simulink model "model3"  (R2024a)
settings: Solver=FixedStepAuto  StartTime=0.0  StopTime=36000  FixedStep=0.1  RelTol=1e-3
settings Model: Creator=rigel  LastModifiedBy=rigel

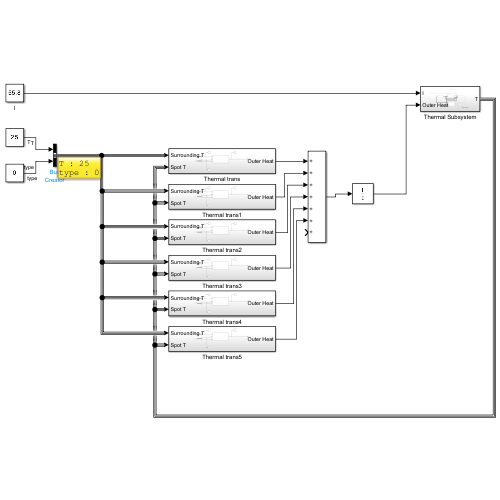
[thumbnail: Simulink's stored preview of the top-level diagram]
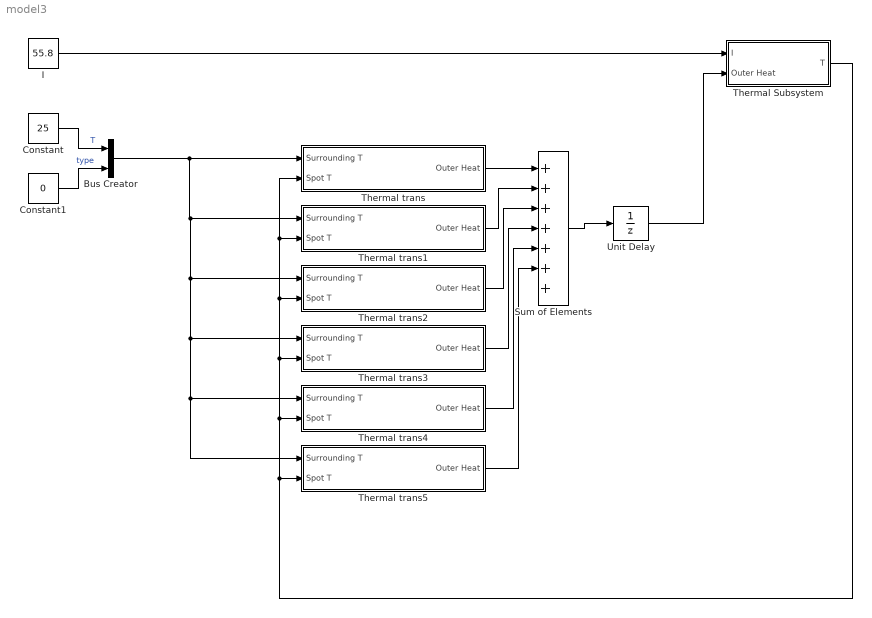
== system model3 ==
  Bus Creator : BusCreator  Inputs=2
  Constant : Constant  Value=25
  Constant1 : Constant  Value=0
  I : Constant  Value=55.8
  Sum of Elements : Sum  Inputs=+++++++
  Thermal Subsystem : Subsystem
  Thermal trans : Subsystem
  Thermal trans1 : Subsystem
  Thermal trans2 : Subsystem
  Thermal trans3 : Subsystem
  Thermal trans4 : Subsystem
  Thermal trans5 : Subsystem
  Unit Delay : UnitDelay  SampleTime=-1  HasFrameUpgradeWarning=on
  wires:
  Thermal Subsystem/1(T) -> Thermal trans/2(Spot T), Thermal trans1/2(Spot T), Thermal trans2/2(Spot T), Thermal trans3/2(Spot T), Thermal trans4/2(Spot T), Thermal trans5/2(Spot T)
  I/1 -> Thermal Subsystem/1(I)
  Unit Delay/1 -> Thermal Subsystem/2(Outer Heat)
  Constant/1 -> Bus Creator/1  "T"
  Constant1/1 -> Bus Creator/2  "type"
  Sum of Elements/1 -> Unit Delay/1
  Thermal trans/1(Outer Heat) -> Sum of Elements/1
  Thermal trans1/1(Outer Heat) -> Sum of Elements/2
  Thermal trans2/1(Outer Heat) -> Sum of Elements/3
  Thermal trans3/1(Outer Heat) -> Sum of Elements/4
  Thermal trans4/1(Outer Heat) -> Sum of Elements/5
  Thermal trans5/1(Outer Heat) -> Sum of Elements/6
  Bus Creator/1 -> Thermal trans5/1(Surrounding T), Thermal trans4/1(Surrounding T), Thermal trans3/1(Surrounding T), Thermal trans2/1(Surrounding T), Thermal trans1/1(Surrounding T), Thermal trans/1(Surrounding T)

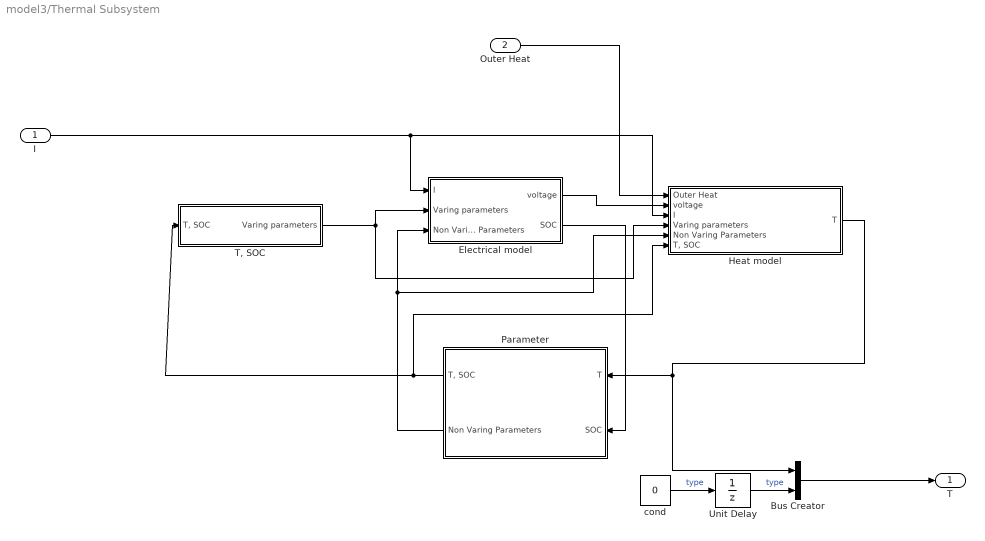
== system model3/Thermal Subsystem ==
  I : Inport
  Outer Heat : Inport  Port=2
  Bus Creator : BusCreator  Inputs=2
  Electrical model : Subsystem
  Heat model : Subsystem
  Parameter : Subsystem
  "T, SOC" : Subsystem
  Unit Delay : UnitDelay  SampleTime=-1  HasFrameUpgradeWarning=on
  cond : Constant  Value=0
  T : Outport
  wires:
  Parameter/2(Non Varing Parameters) -> Electrical model/3(Non Varing Parameters), Heat model/5(Non Varing Parameters)
  "T, SOC"/1(Varing parameters) -> Electrical model/2(Varing parameters), Heat model/4(Varing parameters)
  I/1 -> Heat model/3(I), Electrical model/1(I)
  Electrical model/2(SOC) -> Parameter/2(SOC)
  Electrical model/1(voltage) -> Heat model/2(voltage)
  Parameter/1("T, SOC") -> Heat model/6("T, SOC"), "T, SOC"/1("T, SOC")
  Outer Heat/1 -> Heat model/1(Outer Heat)
  Heat model/1(T) -> Bus Creator/1, Parameter/1(T)
  Bus Creator/1 -> T/1
  cond/1 -> Unit Delay/1  "type"
  Unit Delay/1 -> Bus Creator/2  "type"

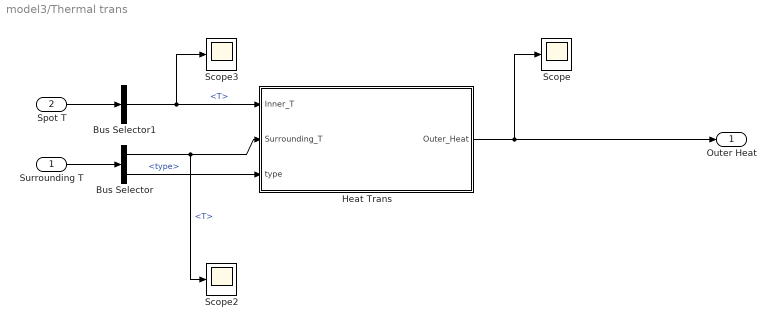
== system model3/Thermal trans ==
  Surrounding T : Inport
  Spot T : Inport  Port=2
  Bus Selector : BusSelector  OutputSignals=T,type
  Bus Selector1 : BusSelector  OutputSignals=T
  Heat Trans : MATLAB Function  TreatAsAtomicUnit=on
  Scope : Scope
  Scope2 : Scope
  Scope3 : Scope
  Outer Heat : Outport
  wires:
  Heat Trans/1(Outer_Heat) -> Scope/1, Outer Heat/1
  Bus Selector/1 -> Scope2/1, Heat Trans/2(Surrounding_T)  "<T>"
  Bus Selector/2 -> Heat Trans/3(type)  "<type>"
  Bus Selector1/1 -> Scope3/1, Heat Trans/1(Inner_T)  "<T>"
  Spot T/1 -> Bus Selector1/1
  Surrounding T/1 -> Bus Selector/1

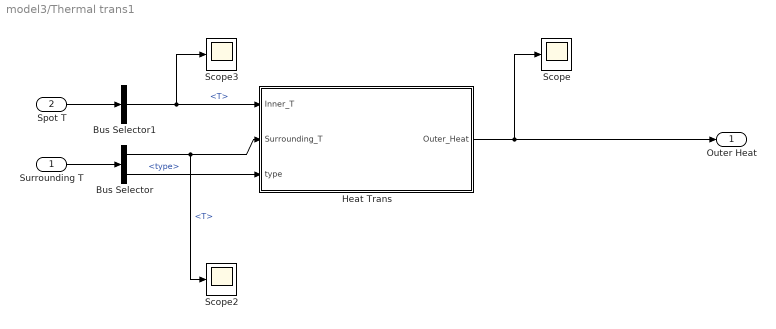
== system model3/Thermal trans1 ==
  Surrounding T : Inport
  Spot T : Inport  Port=2
  Bus Selector : BusSelector  OutputSignals=T,type
  Bus Selector1 : BusSelector  OutputSignals=T
  Heat Trans : MATLAB Function  TreatAsAtomicUnit=on
  Scope : Scope
  Scope2 : Scope
  Scope3 : Scope
  Outer Heat : Outport
  wires:
  Heat Trans/1(Outer_Heat) -> Scope/1, Outer Heat/1
  Bus Selector/1 -> Scope2/1, Heat Trans/2(Surrounding_T)  "<T>"
  Bus Selector/2 -> Heat Trans/3(type)  "<type>"
  Bus Selector1/1 -> Scope3/1, Heat Trans/1(Inner_T)  "<T>"
  Spot T/1 -> Bus Selector1/1
  Surrounding T/1 -> Bus Selector/1

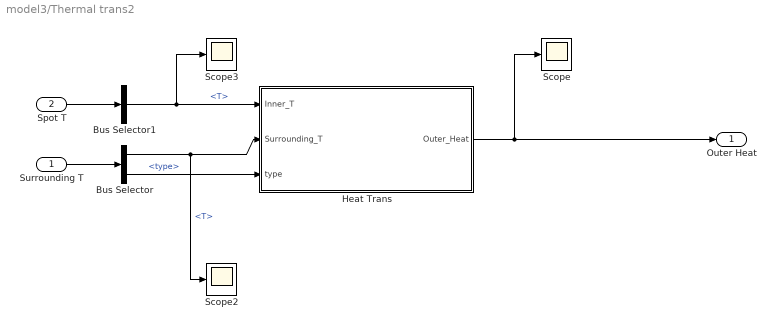
== system model3/Thermal trans2 ==
  Surrounding T : Inport
  Spot T : Inport  Port=2
  Bus Selector : BusSelector  OutputSignals=T,type
  Bus Selector1 : BusSelector  OutputSignals=T
  Heat Trans : MATLAB Function  TreatAsAtomicUnit=on
  Scope : Scope
  Scope2 : Scope
  Scope3 : Scope
  Outer Heat : Outport
  wires:
  Heat Trans/1(Outer_Heat) -> Scope/1, Outer Heat/1
  Bus Selector/1 -> Scope2/1, Heat Trans/2(Surrounding_T)  "<T>"
  Bus Selector/2 -> Heat Trans/3(type)  "<type>"
  Bus Selector1/1 -> Scope3/1, Heat Trans/1(Inner_T)  "<T>"
  Spot T/1 -> Bus Selector1/1
  Surrounding T/1 -> Bus Selector/1

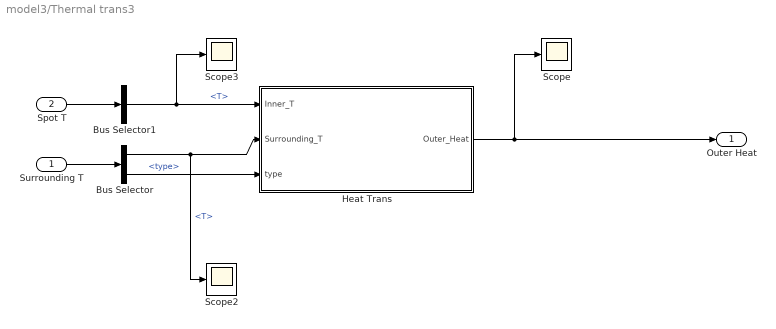
== system model3/Thermal trans3 ==
  Surrounding T : Inport
  Spot T : Inport  Port=2
  Bus Selector : BusSelector  OutputSignals=T,type
  Bus Selector1 : BusSelector  OutputSignals=T
  Heat Trans : MATLAB Function  TreatAsAtomicUnit=on
  Scope : Scope
  Scope2 : Scope
  Scope3 : Scope
  Outer Heat : Outport
  wires:
  Heat Trans/1(Outer_Heat) -> Scope/1, Outer Heat/1
  Bus Selector/1 -> Scope2/1, Heat Trans/2(Surrounding_T)  "<T>"
  Bus Selector/2 -> Heat Trans/3(type)  "<type>"
  Bus Selector1/1 -> Scope3/1, Heat Trans/1(Inner_T)  "<T>"
  Spot T/1 -> Bus Selector1/1
  Surrounding T/1 -> Bus Selector/1

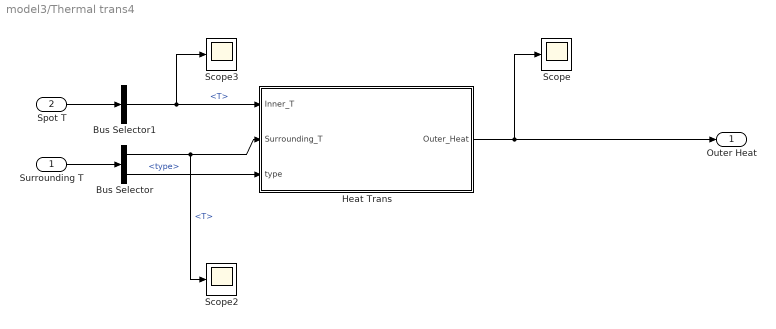
== system model3/Thermal trans4 ==
  Surrounding T : Inport
  Spot T : Inport  Port=2
  Bus Selector : BusSelector  OutputSignals=T,type
  Bus Selector1 : BusSelector  OutputSignals=T
  Heat Trans : MATLAB Function  TreatAsAtomicUnit=on
  Scope : Scope
  Scope2 : Scope
  Scope3 : Scope
  Outer Heat : Outport
  wires:
  Heat Trans/1(Outer_Heat) -> Scope/1, Outer Heat/1
  Bus Selector/1 -> Scope2/1, Heat Trans/2(Surrounding_T)  "<T>"
  Bus Selector/2 -> Heat Trans/3(type)  "<type>"
  Bus Selector1/1 -> Scope3/1, Heat Trans/1(Inner_T)  "<T>"
  Spot T/1 -> Bus Selector1/1
  Surrounding T/1 -> Bus Selector/1

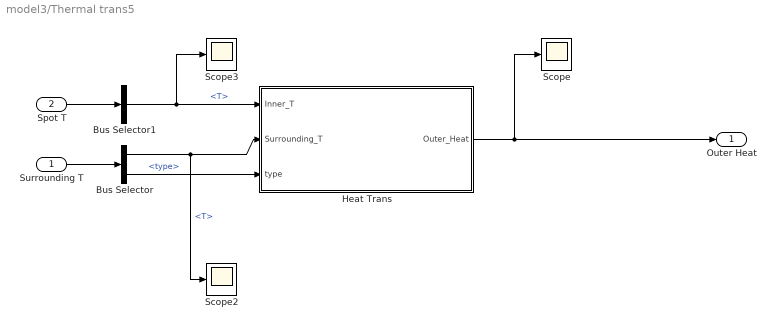
== system model3/Thermal trans5 ==
  Surrounding T : Inport
  Spot T : Inport  Port=2
  Bus Selector : BusSelector  OutputSignals=T,type
  Bus Selector1 : BusSelector  OutputSignals=T
  Heat Trans : MATLAB Function  TreatAsAtomicUnit=on
  Scope : Scope
  Scope2 : Scope
  Scope3 : Scope
  Outer Heat : Outport
  wires:
  Heat Trans/1(Outer_Heat) -> Scope/1, Outer Heat/1
  Bus Selector/1 -> Scope2/1, Heat Trans/2(Surrounding_T)  "<T>"
  Bus Selector/2 -> Heat Trans/3(type)  "<type>"
  Bus Selector1/1 -> Scope3/1, Heat Trans/1(Inner_T)  "<T>"
  Spot T/1 -> Bus Selector1/1
  Surrounding T/1 -> Bus Selector/1

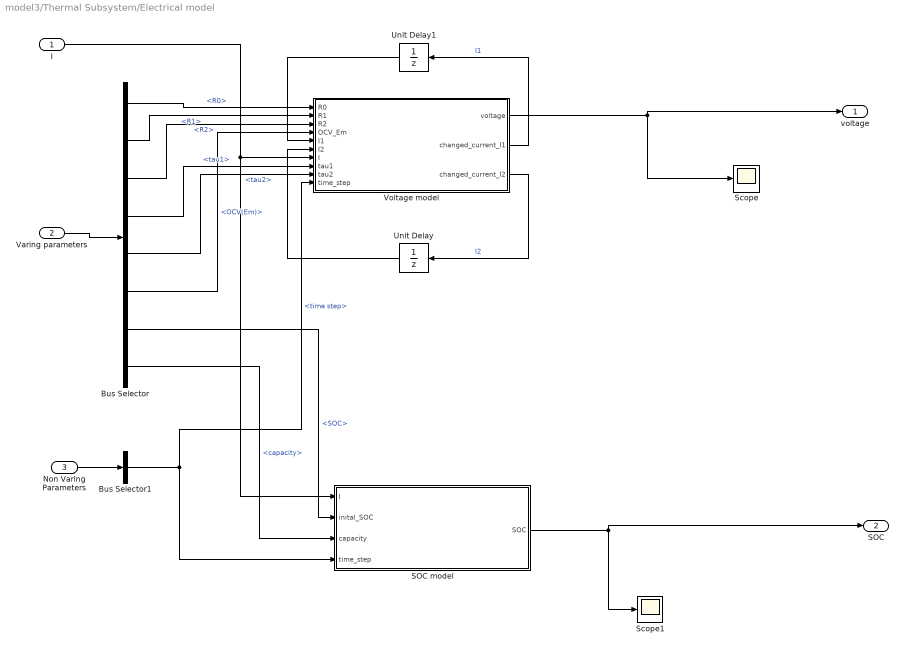
== system model3/Thermal Subsystem/Electrical model ==
  I : Inport
  Varing parameters : Inport  Port=2
  Non Varing Parameters : Inport  Port=3
  Bus Selector : BusSelector  OutputSignals=R0,R1,R2,tau1,tau2,OCV(Em),SOC,capacity
  Bus Selector1 : BusSelector  OutputSignals=time step
  SOC model : MATLAB Function  TreatAsAtomicUnit=on
  Scope : Scope
  Scope1 : Scope
  Unit Delay : UnitDelay  SampleTime=-1  HasFrameUpgradeWarning=on
  Unit Delay1 : UnitDelay  SampleTime=-1  HasFrameUpgradeWarning=on
  Voltage model : MATLAB Function  TreatAsAtomicUnit=on
  voltage : Outport
  SOC : Outport  Port=2
  wires:
  Varing parameters/1 -> Bus Selector/1
  Bus Selector/1 -> Voltage model/1(R0)  "<R0>"
  Bus Selector/2 -> Voltage model/2(R1)  "<R1>"
  Bus Selector/3 -> Voltage model/3(R2)  "<R2>"
  Bus Selector/4 -> Voltage model/8(tau1)  "<tau1>"
  Bus Selector/5 -> Voltage model/9(tau2)  "<tau2>"
  Bus Selector/6 -> Voltage model/4(OCV_Em)  "<OCV(Em)>"
  SOC model/1(SOC) -> SOC/1, Scope1/1
  Voltage model/1(voltage) -> voltage/1, Scope/1
  I/1 -> SOC model/1(I), Voltage model/7(I)
  Voltage model/2(changed_current_I1) -> Unit Delay1/1  "I1"
  Unit Delay1/1 -> Voltage model/5(I1)
  Voltage model/3(changed_current_I2) -> Unit Delay/1  "I2"
  Unit Delay/1 -> Voltage model/6(I2)
  Bus Selector/7 -> SOC model/2(inital_SOC)  "<SOC>"
  Non Varing Parameters/1 -> Bus Selector1/1
  Bus Selector1/1 -> Voltage model/10(time_step), SOC model/4(time_step)  "<time step>"
  Bus Selector/8 -> SOC model/3(capacity)  "<capacity>"

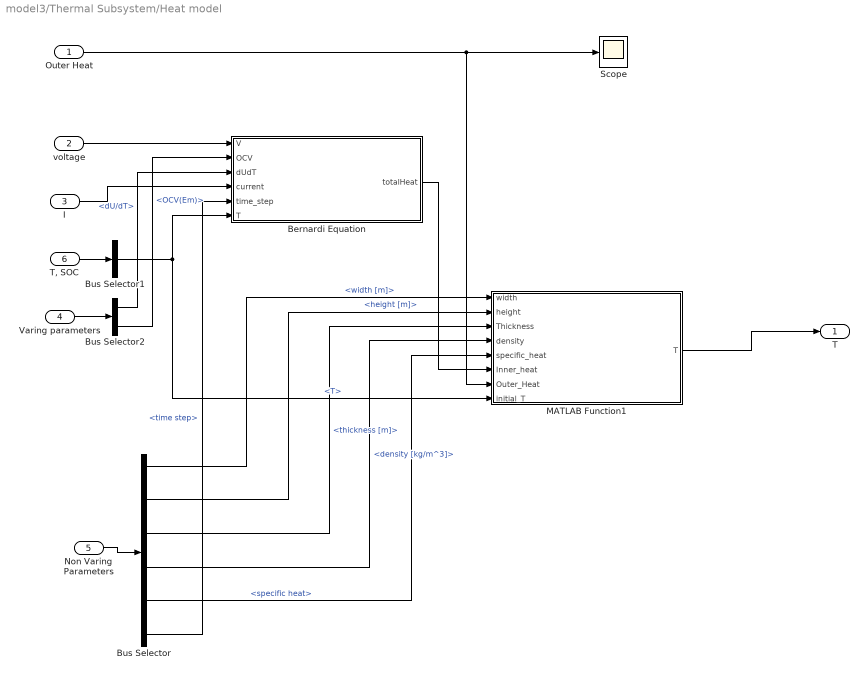
== system model3/Thermal Subsystem/Heat model ==
  Outer Heat : Inport
  voltage : Inport  Port=2
  I : Inport  Port=3
  Varing parameters : Inport  Port=4
  Non Varing Parameters : Inport  Port=5
  "T, SOC" : Inport  Port=6
  Bernardi Equation : MATLAB Function  TreatAsAtomicUnit=on
  Bus Selector : BusSelector  OutputSignals=width [m],height [m],thickness [m],density [kg/m^3],specific heat,time step
  Bus Selector1 : BusSelector  OutputSignals=T
  Bus Selector2 : BusSelector  OutputSignals=dU/dT,OCV(Em)
  MATLAB Function1 : MATLAB Function  TreatAsAtomicUnit=on
  Scope : Scope
  T : Outport
  wires:
  voltage/1 -> Bernardi Equation/1(V)
  MATLAB Function1/1(T) -> T/1
  Bernardi Equation/1(totalHeat) -> MATLAB Function1/6(Inner_heat)
  Non Varing Parameters/1 -> Bus Selector/1
  Bus Selector/1 -> MATLAB Function1/1(width)  "<width [m]>"
  Bus Selector/2 -> MATLAB Function1/2(height)  "<height [m]>"
  Bus Selector/3 -> MATLAB Function1/3(Thickness)  "<thickness [m]>"
  Bus Selector/4 -> MATLAB Function1/4(density)  "<density [kg/m^3]>"
  Bus Selector/5 -> MATLAB Function1/5(specific_heat)  "<specific heat>"
  "T, SOC"/1 -> Bus Selector1/1
  Bus Selector1/1 -> MATLAB Function1/8(initial_T), Bernardi Equation/6(T)  "<T>"
  I/1 -> Bernardi Equation/4(current)
  Varing parameters/1 -> Bus Selector2/1
  Bus Selector2/1 -> Bernardi Equation/3(dUdT)  "<dU/dT>"
  Bus Selector2/2 -> Bernardi Equation/2(OCV)  "<OCV(Em)>"
  Bus Selector/6 -> Bernardi Equation/5(time_step)  "<time step>"
  Outer Heat/1 -> MATLAB Function1/7(Outer_Heat), Scope/1

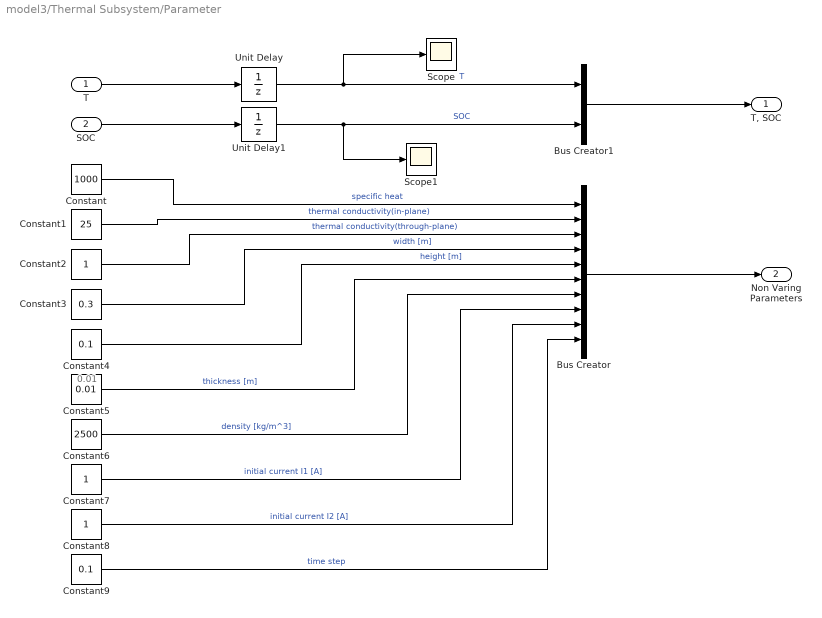
== system model3/Thermal Subsystem/Parameter ==
  note: 0.01
  T : Inport
  SOC : Inport  Port=2
  Bus Creator : BusCreator  Inputs=10
  Bus Creator1 : BusCreator  Inputs=2
  Constant : Constant  Value=1000
  Constant1 : Constant  Value=25
  Constant2 : Constant
  Constant3 : Constant  Value=0.3
  Constant4 : Constant  Value=0.1
  Constant5 : Constant  Value=0.01
  Constant6 : Constant  Value=2500
  Constant7 : Constant
  Constant8 : Constant
  Constant9 : Constant  Value=0.1
  Scope : Scope
  Scope1 : Scope
  Unit Delay : UnitDelay  InitialCondition=25  HasFrameUpgradeWarning=on
  Unit Delay1 : UnitDelay  InitialCondition=1  HasFrameUpgradeWarning=on
  "T, SOC" : Outport
  Non Varing Parameters : Outport  Port=2
  wires:
  Constant2/1 -> Bus Creator/3  "thermal conductivity(through-plane)"
  Constant/1 -> Bus Creator/1  "specific heat"
  Constant8/1 -> Bus Creator/9  "initial current I2 [A]"
  Constant6/1 -> Bus Creator/7  "density [kg/m^3]"
  Constant5/1 -> Bus Creator/6  "thickness [m]"
  Constant1/1 -> Bus Creator/2  "thermal conductivity(in-plane)"
  Constant4/1 -> Bus Creator/5  "height [m]"
  Constant7/1 -> Bus Creator/8  "initial current I1 [A]"
  Constant3/1 -> Bus Creator/4  "width [m]"
  Unit Delay/1 -> Scope/1, Bus Creator1/1  "T"
  Unit Delay1/1 -> Scope1/1, Bus Creator1/2  "SOC"
  T/1 -> Unit Delay/1
  SOC/1 -> Unit Delay1/1
  Bus Creator1/1 -> "T, SOC"/1
  Bus Creator/1 -> Non Varing Parameters/1
  Constant9/1 -> Bus Creator/10  "time step"

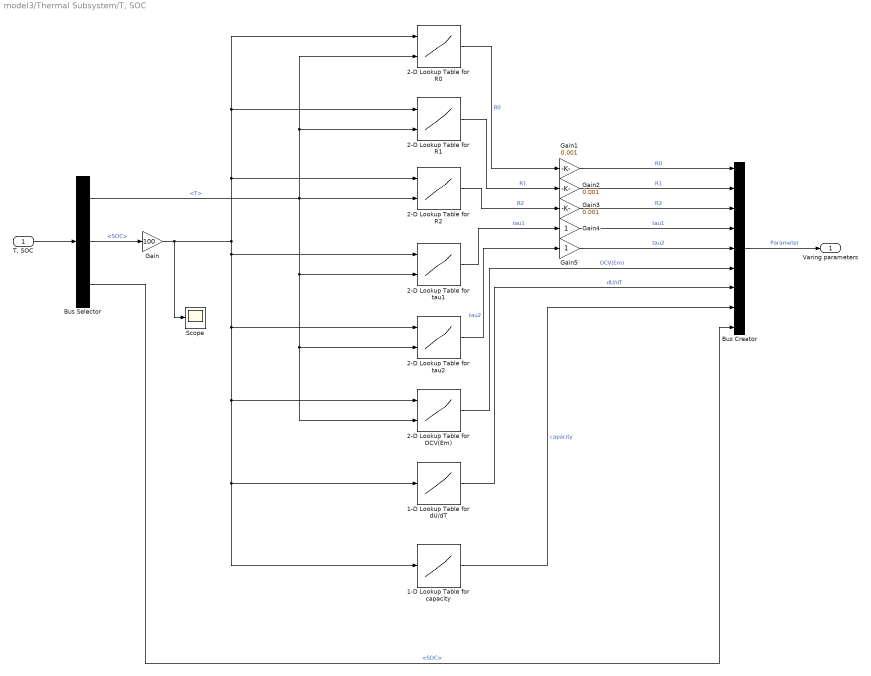
== system model3/Thermal Subsystem/T, SOC ==
  "T, SOC" : Inport
  1-D Lookup Table for capacity : Lookup_n-D  NumberOfTableDimensions=1  BreakpointsForDimension1=[5;15;25;35;45]  Table=[51.8;54.3;55.8;57.2;57.3]  InternalRulePriority=Speed  RndMeth=Simplest
  1-D Lookup Table for dU/dT : Lookup_n-D  NumberOfTableDimensions=1  BreakpointsForDimension1=[0 10 20 30 40 50 60 70 80 90 100]  Table=[-0.0004 -9e-05 -3e-05 9e-05 0.00016 9e-05 5e-05 5e-05 6e-05 9e-05 8e-05]  InternalRulePriority=Speed  RndMeth=Simplest
  2-D Lookup Table for OCV(Em) : Lookup_n-D  BreakpointsForDimension1=[0;2.5;4.987882;7.488427;9.988971;14.98952;19.99007;24.99062;29.99118;34.99173;39.99229;44.99284;49.9934;54.99394;59.99449;64.99504;69.99559;74.99614;79.99669;84.99724;89.99779;92.49834;94.9989;97.49945;100]  BreakpointsForDimension2=[5 15 25 35 45]  Table=[3.41 3.37 3.23 3.23 3.23;3.43 3.4 3.36 3.36 3.36;3.45 3.42 3.4 3.41 3.41;3.48 3.44 3.42 3.43 3.43;3.51 3.47 3.44 3.45 3.45;3.55 3.52 3.5 3.5 3.5;3.58 3.56 3.54 3.55 3.55;3.6 3.59 3.58 3.58 3.58;3.61 3.61 3.6 3.61 3.61;3.63 3.63 3.62 3.62 3.62;3.65 3.65 3.64 3.64 3.64;3.68 3.67 3.66 3.67 3.67;3.72 3.71 3.7 3.7 3.7;3.78 3.77 3.75 3.76 3.76;3.83 3.82 3.81 3.81 3.81;3.87 3.86 3.85 3.86 3.86;3.91 3.9 3.89 3.9 3.9;3.94 3.94 3.93 3.94 3.94;4 3.99 3.98 3.99 3.99;4.04 4.04 4.03 4.04 4.04;4.07 4.08 4.07 4.08 4.08;4.08 4.09 4.09 4.09 4.09;4.1 4.1 4.1 4.11 4.11;4.12 4.13 4.13 4.14 4.14;4.17 4.18 4.18 4.19 4.19]  InternalRulePriority=Speed  RndMeth=Simplest
      settings: InputPortMap=u0,u1
  2-D Lookup Table for R0 : Lookup_n-D  BreakpointsForDimension1=[4.987882;7.488427;9.988971;14.98952;19.99007;24.99062;29.99118;34.99173;39.99229;44.99284;49.9934;54.99394;59.99449;64.99504;69.99559;74.99614;79.99669;84.99724;89.99779;92.49834;94.9989;97.49945;100]  BreakpointsForDimension2=[5 15 25 35 45]  Table=[2.5 1.660027 1.399329 1 0.85;2.5 1.567803 1.309628 0.95 0.8;2 1.512469 1.237868 0.9 0.75;2 1.383279 1.130227 0.8 0.7;2 1.291108 1.058467 0.75 0.7;1.75 1.235729 1 0.75 0.65;1.75 1.217285 0.95 0.75 0.65;1.75 1.198842 0.95 0.75 0.65;1.75 1.180398 0.95 0.75 0.65;1.75 1.161954 0.95 0.75 0.65;1.75 1.161954 0.95 0.75 0.65;1.5 1.2 0.95 0.7 0.65;1.5 1.2 0.95 0.7 0.65;1.5 1.2 0.95 0.7 0.65;1.5 1.2 0.95 0.7 0.65;1.5 1.2 0.95 0.7 0.65;1.5 1.2 0.95 0.7 0.65;1.75 1.2 0.95 0.75 0.65;1.75 1.180398 0.95 0.75 0.65;1.75 1.198842 0.95 0.75 0.65;2 1.217353 1 0.75 0.65;2 1.235798 1 0.75 0.65;2 1.235798 1 0.75 0.65]  InternalRulePriority=Speed  RndMeth=Simplest
      settings: InputPortMap=u0,u1
  2-D Lookup Table for R1 : Lookup_n-D  BreakpointsForDimension1=[4.987882;7.488427;9.988971;14.98952;19.99007;24.99062;29.99118;34.99173;39.99229;44.99284;49.9934;54.99394;59.99449;64.99504;69.99559;74.99614;79.99669;84.99724;89.99779;92.49834;94.9989;97.49945;100]  BreakpointsForDimension2=[5 15 25 35 45]  Table=[1.343459 1 0.95 0.55 0.4;0.95 0.65 0.65 0.55 0.4;0.7 0.5 0.5 0.45 0.4;0.45 0.4 0.4 0.35 0.35;0.45 0.4 0.4 0.3 0.3;0.4 0.35 0.4 0.3 0.3;0.4 0.4 0.4 0.3 0.3;0.4 0.3 0.4 0.3 0.3;0.35 0.3 0.4 0.3 0.3;0.35 0.3 0.4 0.3 0.3;0.45 0.35 0.4 0.3 0.3;0.5 0.45 0.45 0.35 0.3;0.55 0.5 0.45 0.35 0.3;0.45 0.4 0.4 0.35 0.35;0.45 0.4 0.4 0.35 0.35;0.45 0.4 0.4 0.35 0.3;0.5 0.4 0.4 0.35 0.3;0.45 0.4 0.35 0.25 0.25;0.4 0.35 0.35 0.25 0.25;0.4 0.35 0.35 0.3 0.25;0.45 0.4 0.3 0.25 0.25;0.45 0.45 0.35 0.35 0.25;0.5 0.45 0.4 0.35 0.3]  InternalRulePriority=Speed  RndMeth=Simplest
      settings: InputPortMap=u0,u1
  2-D Lookup Table for R2 : Lookup_n-D  BreakpointsForDimension1=[4.987882;7.488427;9.988971;14.98952;19.99007;24.99062;29.99118;34.99173;39.99229;44.99284;49.9934;54.99394;59.99449;64.99504;69.99559;74.99614;79.99669;84.99724;89.99779;92.49834;94.9989;97.49945;100]  BreakpointsForDimension2=[5 15 25 35 45]  Table=[11.25 10 8 6.3 5.062057;4 3.773492 4.3 2.7 1.418744;3 1.926279 2.088626 1.5 1;2.75 1.741972 1.371574 0.8 0.65;2.5 1.58323 1.235492 0.8 0.65;2 1.585742 1.227908 0.8 0.65;1.75 1.41798 1.3 0.9 0.65;1.75 1.19079 1.090479 0.9 0.65;1.5 1 0.9 0.7 0.7;1.5 0.9 0.9 0.7 0.6;1.5 0.9 0.9 0.7 0.6;1.5 0.9 0.9 0.7 0.6;1.5 1 1 0.8 0.65;1.504995 1.233499 1.1 0.9 0.75;1.47432 1.196612 1 0.8 0.7;1.5 1.138683 0.95 0.75 0.65;1.25 1 0.9 0.7 0.55;1.25 1 0.85 0.6 0.45;1.25 0.9 0.7 0.55 0.4;1 0.8 0.75 0.5 0.4;0.9 0.7 0.6 0.4 0.3;0.9 0.6 0.55 0.4 0.3;1 0.7 0.6 0.4 0.35]  InternalRulePriority=Speed  RndMeth=Simplest
      settings: InputPortMap=u0,u1
  2-D Lookup Table for tau1 : Lookup_n-D  BreakpointsForDimension1=[4.987882;7.488427;9.988971;14.98952;19.99007;24.99062;29.99118;34.99173;39.99229;44.99284;49.9934;54.99394;59.99449;64.99504;69.99559;74.99614;79.99669;84.99724;89.99779;92.49834;94.9989;97.49945;100]  BreakpointsForDimension2=[5 15 25 35 45]  Table=[1.15 1.5 1.96 3.39 3.09;1.25 1.9 2.8 5.27 3.89;1.6 2.3 3.03 5.23 4.07;2.15 3.6 3.65 4.14 4.77;3.35 5.4 5.35 4.55 4.53;3.85 4.1 4.83 3.83 3.53;4.35 6.4 4.6 5.36 3.61;5.15 4.1 4.45 3.75 3.21;4.3 4 5.49 4.61 3.54;3.65 4.3 3.94 3.53 3.71;4.4 4.1 5.2 3.76 2.99;4.55 5.1 5.38 3.7 3.53;4.7 5.8 4.82 4.14 3.43;3.8 4.3 3.59 3.48 4.16;3.7 4.5 4.02 4.38 4.31;3.95 4.4 4.67 4.46 4.07;4.9 4.7 4.09 3.92 3.73;4.5 4.4 4.26 3.1 2.93;3.5 4.4 4.47 3.66 3.47;3.8 3.6 4.29 3.85 2.77;3.5 4.6 3.44 2.98 2.89;3.45 4.8 3.92 4.27 3.32;3.4 4.2 4.42 4.16 3.92]  InternalRulePriority=Speed  RndMeth=Simplest
      settings: InputPortMap=u0,u1
  2-D Lookup Table for tau2 : Lookup_n-D  BreakpointsForDimension1=[4.987882;7.488427;9.988971;14.98952;19.99007;24.99062;29.99118;34.99173;39.99229;44.99284;49.9934;54.99394;59.99449;64.99504;69.99559;74.99614;79.99669;84.99724;89.99779;92.49834;94.9989;97.49945;100]  BreakpointsForDimension2=[5 15 25 35 45]  Table=[185 300 300 93.67 300;75.3 91.2 148.77 105.74 77.83;67.8 53.3 66.88 56.32 53.02;85.4 70.7 59.61 43.37 45.34;86.5 85.4 71.75 54.67 41.7;78.9 75.8 71.19 50.7 40.55;71.8 87.8 71.96 73.22 46.89;66.1 60.7 63.92 57.62 54.37;52.2 52.1 64.06 53.52 48.88;44.6 47.1 47.41 40.53 42.49;41.1 37.4 46.1 35.98 35.33;36.8 31.7 31.79 22.48 20.07;46.1 45.9 37.76 36.57 27;47.9 46.8 41.38 39.18 38.88;49.4 49.4 46.03 44.18 41.55;49.3 48.9 49.79 43.32 38.38;52.3 46.5 43.5 38.44 34.2;53.4 49.7 46.26 35.85 31.25;52.6 54.4 51.32 46.11 41.98;49.6 44.3 54.68 46.3 43.67;36.3 40.6 33.94 25.83 34.83;31.6 33.5 27.37 26.04 19.14;30.3 31.5 29.11 25.72 22.48]  InternalRulePriority=Speed  RndMeth=Simplest
      settings: InputPortMap=u0,u1
  Bus Creator : BusCreator  Inputs=9
  Bus Selector : BusSelector  OutputSignals=T,SOC,SOC
  Gain : Gain  Gain=100
  Gain1 : Gain  Gain=0.001
  Gain2 : Gain  Gain=0.001
  Gain3 : Gain  Gain=0.001
  Gain4 : Gain
  Gain5 : Gain
  Scope : Scope
  Varing parameters : Outport
  wires:
  2-D Lookup Table for OCV(Em)/1 -> Bus Creator/6  "OCV(Em)"
  2-D Lookup Table for tau2/1 -> Gain5/1  "tau2"
  2-D Lookup Table for R2/1 -> Gain3/1  "R2"
  2-D Lookup Table for tau1/1 -> Gain4/1  "tau1"
  2-D Lookup Table for R0/1 -> Gain1/1  "R0"
  2-D Lookup Table for R1/1 -> Gain2/1  "R1"
  Bus Creator/1 -> Varing parameters/1  "Parameter"
  1-D Lookup Table for dU/dT/1 -> Bus Creator/7  "dU/dT"
  "T, SOC"/1 -> Bus Selector/1
  Bus Selector/1 -> 2-D Lookup Table for OCV(Em)/2, 2-D Lookup Table for tau2/2, 2-D Lookup Table for tau1/2, 2-D Lookup Table for R2/2, 2-D Lookup Table for R1/2, 2-D Lookup Table for R0/2  "<T>"
  Bus Selector/3 -> Bus Creator/9  "<SOC>"
  Bus Selector/2 -> Gain/1  "<SOC>"
  Gain/1 -> 2-D Lookup Table for R1/1, 2-D Lookup Table for R0/1, 2-D Lookup Table for R2/1, 2-D Lookup Table for tau2/1, 2-D Lookup Table for OCV(Em)/1, 1-D Lookup Table for dU/dT/1, 1-D Lookup Table for capacity/1, 2-D Lookup Table for tau1/1, Scope/1
  1-D Lookup Table for capacity/1 -> Bus Creator/8  "capacity"
  Gain1/1 -> Bus Creator/1  "R0"
  Gain2/1 -> Bus Creator/2  "R1"
  Gain3/1 -> Bus Creator/3  "R2"
  Gain4/1 -> Bus Creator/4  "tau1"
  Gain5/1 -> Bus Creator/5  "tau2"

== matlab function model3/Thermal trans4/Heat Trans ==
  data: Inner_T input; Outer_Heat output; Surrounding_T input; type input
function Outer_Heat = fcn(Inner_T, Surrounding_T, type)
%#codegen
% Inputs
%   Inner_T        : 내부 온도 (scalar)
%   Surrounding    : struct with fields
%       .T         : 주변 온도
%       .mode      : 0 = conduction, 1 = convection

k = 1;    % 열전도도 (W/(m·K))
A = 0.01;    % 면적 (m^2)
L = 0.1;    % 길이 (m)
h = 1;    % 대류 열전달계수 (W/(m^2·K))

G_cond = k * A / L;      % 전도 전도도 (W/K)
G_conv = h * A;          % 대류 전도도   (W/K)

if type == 0
    % 전도
    % q = G_cond * (ΔT)
    Outer_Heat = - G_cond * (Inner_T - Surrounding_T);
elseif type == 1
    % 대류
    % q = G_conv * (ΔT)
    Outer_Heat = - G_conv * (Inner_T - Surrounding_T);
else
    % 정의되지 않은 모드일 때
    Outer_Heat = 0;
end

== matlab function model3/Thermal trans5/Heat Trans ==
  data: Inner_T input; Outer_Heat output; Surrounding_T input; type input
function Outer_Heat = fcn(Inner_T, Surrounding_T, type)
%#codegen
% Inputs
%   Inner_T        : 내부 온도 (scalar)
%   Surrounding    : struct with fields
%       .T         : 주변 온도
%       .mode      : 0 = conduction, 1 = convection

k = 1;    % 열전도도 (W/(m·K))
A = 0.01;    % 면적 (m^2)
L = 0.1;    % 길이 (m)
h = 1;    % 대류 열전달계수 (W/(m^2·K))

G_cond = k * A / L;      % 전도 전도도 (W/K)
G_conv = h * A;          % 대류 전도도   (W/K)

if type == 0
    % 전도
    % q = G_cond * (ΔT)
    Outer_Heat = - G_cond * (Inner_T - Surrounding_T);
elseif type == 1
    % 대류
    % q = G_conv * (ΔT)
    Outer_Heat = - G_conv * (Inner_T - Surrounding_T);
else
    % 정의되지 않은 모드일 때
    Outer_Heat = 0;
end

== matlab function model3/Thermal trans/Heat Trans ==
  data: Inner_T input; Outer_Heat output; Surrounding_T input; type input
function Outer_Heat = fcn(Inner_T, Surrounding_T, type)
%#codegen
% Inputs
%   Inner_T        : 내부 온도 (scalar)
%   Surrounding    : struct with fields
%       .T         : 주변 온도
%       .mode      : 0 = conduction, 1 = convection

k = 1;    % 열전도도 (W/(m·K))
A = 0.01;    % 면적 (m^2)
L = 0.1;    % 길이 (m)
h = 1;    % 대류 열전달계수 (W/(m^2·K))

G_cond = k * A / L;      % 전도 전도도 (W/K)
G_conv = h * A;          % 대류 전도도   (W/K)

if type == 0
    % 전도
    % q = G_cond * (ΔT)
    Outer_Heat = - G_cond * (Inner_T - Surrounding_T);
elseif type == 1
    % 대류
    % q = G_conv * (ΔT)
    Outer_Heat = - G_conv * (Inner_T - Surrounding_T);
else
    % 정의되지 않은 모드일 때
    Outer_Heat = 0;
end

== matlab function model3/Thermal Subsystem/Electrical model/SOC model ==
  data: SOC output; I input; inital_SOC input; capacity input; time_step input
function SOC = fcn(I, inital_SOC, capacity, time_step)
    % Cn = 55.8 * 3600;
    SOC = inital_SOC - (I * time_step / (capacity * 3600));
end

== matlab function model3/Thermal Subsystem/Electrical model/Voltage model ==
  data: R0 input; voltage output; R1 input; R2 input; OCV_Em input; I1 input; I2 input; I input; changed_current_I1 output; changed_current_I2 output; tau1 input; tau2 input; time_step input
function [voltage, changed_current_I1, changed_current_I2] = fcn(R0, R1, R2, OCV_Em, I1, I2, I, tau1, tau2, time_step)
    persistent state_I1 state_I2

    if isempty(state_I1) || isempty(state_I2)
        state_I1 = 0;
        state_I2 = 0;
    else
        state_I1 = I1 * exp(-time_step/tau1) + (1 - exp(-time_step/tau1)) * I;
        state_I2 = I2 * exp(-time_step/tau2) + (1 - exp(-time_step/tau2)) * I;
    end

    voltage = OCV_Em - R0 * I - R1 * state_I1 - R2 * state_I2;
    
    changed_current_I1 = state_I1;
    changed_current_I2 = state_I2;
end

== matlab function model3/Thermal Subsystem/Heat model/Bernardi Equation ==
  data: V input; OCV input; dUdT input; current input; time_step input; T input; totalHeat output
function totalHeat  = fcn(V, OCV, dUdT, current, time_step, T)
    revHeat = current * (T + 273.15) * dUdT;
    irrHeat = current * (OCV - V);
    totalHeat = (-revHeat + irrHeat) * time_step;
end

== matlab function model3/Thermal Subsystem/Heat model/MATLAB Function1 ==
  data: width input; T output; height input; Thickness input; density input; specific_heat input; Inner_heat input; Outer_Heat input; initial_T input
function T = fcn(width, height, Thickness, density, specific_heat, Inner_heat, Outer_Heat, initial_T)
    volume = width * height * Thickness;
    mass = volume * density;
    delta_T = (Inner_heat + Outer_Heat) / (mass * specific_heat);
    T = initial_T + delta_T;
end

== matlab function model3/Thermal trans1/Heat Trans ==
  data: Inner_T input; Outer_Heat output; Surrounding_T input; type input
function Outer_Heat = fcn(Inner_T, Surrounding_T, type)
%#codegen
% Inputs
%   Inner_T        : 내부 온도 (scalar)
%   Surrounding    : struct with fields
%       .T         : 주변 온도
%       .mode      : 0 = conduction, 1 = convection

k = 1;    % 열전도도 (W/(m·K))
A = 0.01;    % 면적 (m^2)
L = 0.1;    % 길이 (m)
h = 1;    % 대류 열전달계수 (W/(m^2·K))

G_cond = k * A / L;      % 전도 전도도 (W/K)
G_conv = h * A;          % 대류 전도도   (W/K)

if type == 0
    % 전도
    % q = G_cond * (ΔT)
    Outer_Heat = - G_cond * (Inner_T - Surrounding_T);
elseif type == 1
    % 대류
    % q = G_conv * (ΔT)
    Outer_Heat = - G_conv * (Inner_T - Surrounding_T);
else
    % 정의되지 않은 모드일 때
    Outer_Heat = 0;
end

== matlab function model3/Thermal trans2/Heat Trans ==
  data: Inner_T input; Outer_Heat output; Surrounding_T input; type input
function Outer_Heat = fcn(Inner_T, Surrounding_T, type)
%#codegen
% Inputs
%   Inner_T        : 내부 온도 (scalar)
%   Surrounding    : struct with fields
%       .T         : 주변 온도
%       .mode      : 0 = conduction, 1 = convection

k = 1;    % 열전도도 (W/(m·K))
A = 0.01;    % 면적 (m^2)
L = 0.1;    % 길이 (m)
h = 1;    % 대류 열전달계수 (W/(m^2·K))

G_cond = k * A / L;      % 전도 전도도 (W/K)
G_conv = h * A;          % 대류 전도도   (W/K)

if type == 0
    % 전도
    % q = G_cond * (ΔT)
    Outer_Heat = - G_cond * (Inner_T - Surrounding_T);
elseif type == 1
    % 대류
    % q = G_conv * (ΔT)
    Outer_Heat = - G_conv * (Inner_T - Surrounding_T);
else
    % 정의되지 않은 모드일 때
    Outer_Heat = 0;
end

== matlab function model3/Thermal trans3/Heat Trans ==
  data: Inner_T input; Outer_Heat output; Surrounding_T input; type input
function Outer_Heat = fcn(Inner_T, Surrounding_T, type)
%#codegen
% Inputs
%   Inner_T        : 내부 온도 (scalar)
%   Surrounding    : struct with fields
%       .T         : 주변 온도
%       .mode      : 0 = conduction, 1 = convection

k = 1;    % 열전도도 (W/(m·K))
A = 0.01;    % 면적 (m^2)
L = 0.1;    % 길이 (m)
h = 1;    % 대류 열전달계수 (W/(m^2·K))

G_cond = k * A / L;      % 전도 전도도 (W/K)
G_conv = h * A;          % 대류 전도도   (W/K)

if type == 0
    % 전도
    % q = G_cond * (ΔT)
    Outer_Heat = - G_cond * (Inner_T - Surrounding_T);
elseif type == 1
    % 대류
    % q = G_conv * (ΔT)
    Outer_Heat = - G_conv * (Inner_T - Surrounding_T);
else
    % 정의되지 않은 모드일 때
    Outer_Heat = 0;
end
